simulink model "Model_Platform"  (R2018a)
settings: Solver=ode1  StartTime=0.0  StopTime=inf  FixedStep=0.001  RelTol=1e-3  EnableMultiTasking=on
PreLoadFcn:
  | ;HLABlocksetInit;;HLABlocksetInit;;HLABlocksetInit;
PostLoadFcn:
  | ;set_param(gcs,'PostCodeGenCommand', 'rtw_defines(buildInfo)');;set_param(gcs,'PostCodeGenCommand', 'rtw_defines(buildInfo)');;set_param(gcs,'PostCodeGenCommand', 'rtw_defines(buildInfo)');
undefined symbols (not defined in the file or in its folder): eng_speed, Heading_init, inertiaLateral, Joystick, Newton, omega_engine, omega_max, omega_wheel, Para, radiusWheel, Raphson, Standard_Devices, torque, Torque_lost, Torque_lost_wheel, X_init, Y_init, Z_init
libraries: simulink x26, dspnetwork x4, rtwinlib x2, PC_Simulator_Lib x2, vrlib x1
(part 1 of 4)
settings Model: ExtModeTrigDuration=1000001  Creator=Mohamed  LastModifiedBy=mario.franke
settings DataIOCC: LimitDataPoints=on  SaveFormat=Array  SignalLoggingSaveFormat=ModelDataLogs  ReturnWorkspaceOutputs=on
settings OptimizationCC: ExpressionDepthLimit=2147483647  LifeSpan=inf
settings DebuggingCC: ReadBeforeWriteMsg=DisableAll  WriteAfterWriteMsg=DisableAll  WriteAfterReadMsg=DisableAll  UnderspecifiedInitializationDetection=Classic  MergeDetectMultiDrivingBlocksExec=none  SolverPrmCheckMsg=warning  MultiTaskDSMMsg=none  MultiTaskRateTransMsg=warning  IntegerOverflowMsg=none  StateNameClashWarn=warning  SFUnexpectedBacktrackingDiag=warning  SFNoUnconditionalDefaultTransitionDiag=warning  SFExecutionAtInitializationDiag=none  IntegerSaturationMsg=none
settings HardwareCC: ProdBitPerPointer=32  ProdBitPerSizeT=32  ProdBitPerPtrDiffT=32  ProdLargestAtomicFloat=None  ProdWordSize=32  ProdHWDeviceType=Generic->32-bit x86 compatible
settings ModelReferenceCC: UpdateModelReferenceTargets=IfOutOfDate  PropagateSignalLabelsOutOfModel=off
settings SFSimCC: SFSimEcho=off
settings RTWCC: PostCodeGenCommand=rtw_defines(buildInfo)  Description=Generic Real-Time Target  RTWCompilerOptimization=on
settings CodeAppCC: MaxIdLength=95  StateflowObjectComments=on
settings GRTTargetCC: TargetLangStandard=C89/C90 (ANSI)  GeneratePreprocessorConditionals=Disable all
settings ConfigComp: CovMetricSettings=dw  CovHtmlReporting=on  CovSaveCumulativeToWorkspaceVar=on  CovSaveSingleToWorkspaceVar=on  CovExternalEMLEnable=off
settings SimscapeCC: SimscapeNormalizeSystem=off
settings ConfigurationSet: Description=SimMechanics 2G

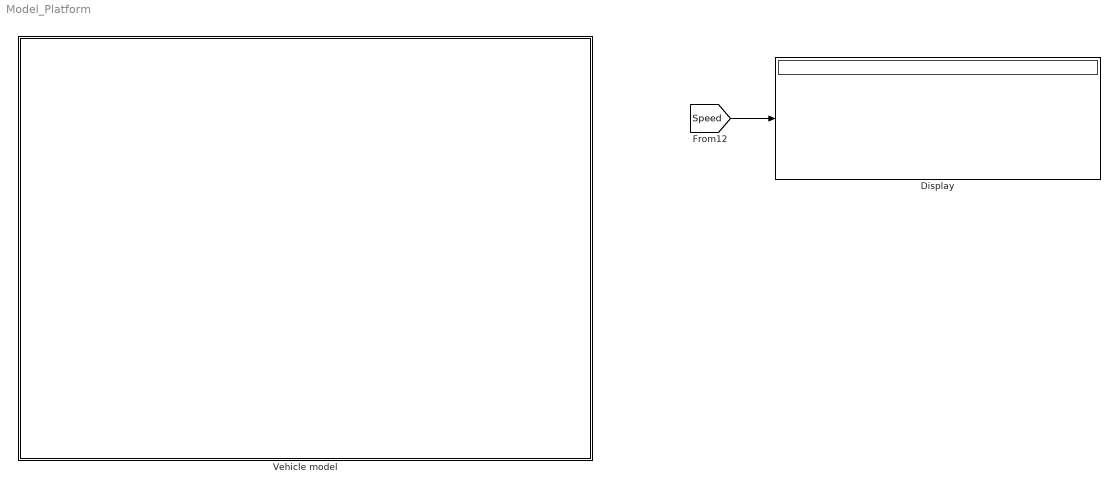
== system Model_Platform ==
  Display : Display
      settings: Format=bank
  Vehicle model : Subsystem
      mask Display: image(imread('Image.jpg'))
  wires:
  [Speed] -> Display/1

== system Model_Platform/Vehicle model ==
  Bus Creator : BusCreator  Inputs=3
  Comunication_with_visualisation_normal_mode1 : Subsystem  AncestorBlock=PC_Simulator_Lib/Comunication_with_visualisation_normal_mode
  Display : Display
      settings: Format=bank
  Drive_Train : Subsystem  AncestorBlock=PC_Simulator_Lib/Drive_Train
  HMI_Realtime_normal_mode : Subsystem  AncestorBlock=PC_Simulator_Lib/HMI_Realtime_normal_mode
  Remaining Computation Time (must be positive) : Scope  Commented=on
  Timer for Real-Time : S-Function  FunctionName=sfun_rttime  Parameters=1  SFunctionDeploymentMode=off  EnableBusSupport=off
  Vehicle dynamics : Subsystem  AncestorBlock=PC_Simulator_Lib/Vehicle dynamics
  wires:
  Drive_Train/1(Drive_Train) -> Bus Creator/2
  Bus Creator/1 -> HMI_Realtime_normal_mode/1(feedback), Drive_Train/1(feedback), Comunication_with_visualisation_normal_mode1/1(FeedBack), Vehicle dynamics/1(Feedback)
  Vehicle dynamics/1(Vehicle_Dynamics) -> Bus Creator/3
  Timer for Real-Time/1 -> Remaining Computation Time (must be positive)/1
  [Speed] -> Display/1
  HMI_Realtime_normal_mode/1(Driver_Interface) -> Bus Creator/1

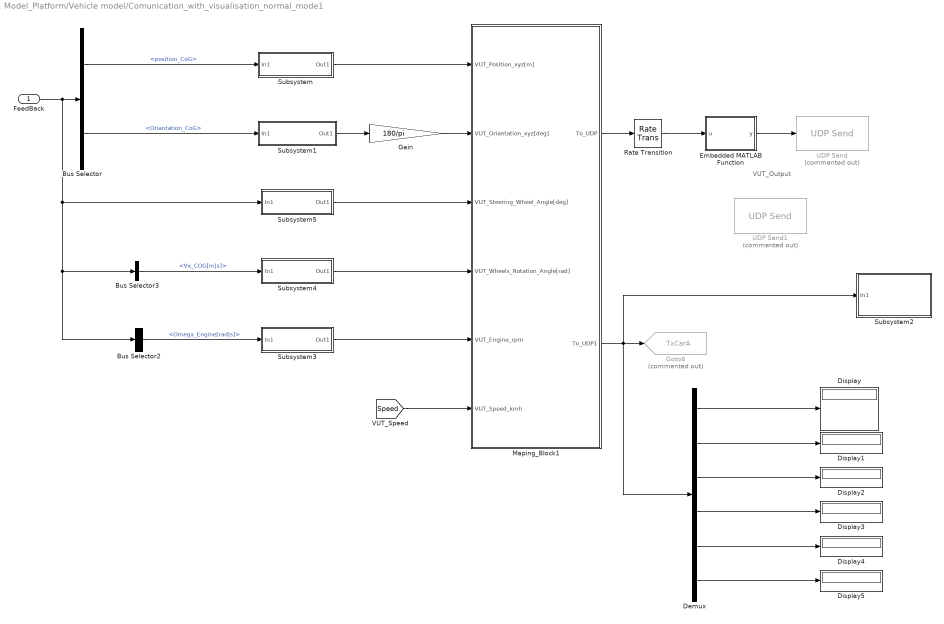
== system Model_Platform/Vehicle model/Comunication_with_visualisation_normal_mode1 ==
  note: VUT_Output
  FeedBack : Inport
  Bus Selector : BusSelector  OutputSignals=Vehicle_Dynamics.position_CoG,Vehicle_Dynamics.Oriantation_CoG
  Bus Selector2 : BusSelector  OutputSignals=Drive_Train.Omega_Engine[rad|s]
  Bus Selector3 : BusSelector  OutputSignals=Vehicle_Dynamics.Vx_COG[m|s]
  Demux : Demux  Outputs=6
  Display{,1..5} (6 alike) : Display
  Embedded MATLAB Function : MATLAB Function  TreatAsAtomicUnit=on
  Gain : Gain  Gain=180/pi
  Goto6 : Goto  Commented=on  GotoTag=TxCarA  TagVisibility=global
  Maping_Block1 : Subsystem
  Rate Transition : RateTransition
  Subsystem : Subsystem
  Subsystem1 : Subsystem
  Subsystem2 : Subsystem  TreatAsAtomicUnit=on  SystemSampleTime=1/20
  Subsystem3 : Subsystem
  Subsystem4 : Subsystem
  Subsystem5 : Subsystem
  UDP Send : dspnetwork/UDP Send  Commented=on  remoteURL='169.254.83.115'  remotePort=15005  localURL='0.0.0.0'  localPortSource=Specify via dialog  localPort=-1  sampletime=-1  blockPlatform=[]  separateLengthPort=0
      settings: SourceProductName=DSP System Toolbox  SourceProductBaseCode=DS
  UDP Send1 : dspnetwork/UDP Send  Commented=on  remoteURL='131.234.86.53'  remotePort=14000  localURL='0.0.0.0'  localPortSource=Specify via dialog  localPort=-1  sampletime=-1  blockPlatform=[]  separateLengthPort=0
      settings: SourceProductName=DSP System Toolbox  SourceProductBaseCode=DS
  wires:
  Embedded MATLAB Function/1(y) -> UDP Send/1
  Bus Selector/2 -> Subsystem1/1(In1)  "<Oriantation_CoG>"
  Bus Selector/1 -> Subsystem/1(In1)  "<position_CoG>"
  Subsystem1/1(Out1) -> Gain/1
  Gain/1 -> Maping_Block1/2(VUT_Oriantation_xyz[deg])
  Maping_Block1/1(To_UDP) -> Rate Transition/1
  Subsystem3/1(Out1) -> Maping_Block1/5(VUT_Engine_rpm)
  Bus Selector3/1 -> Subsystem4/1(In1)  "<Vx_COG[m|s]>"
  Subsystem4/1(Out1) -> Maping_Block1/4(VUT_Wheels_Rotation_Angle[rad])
  FeedBack/1 -> Bus Selector2/1, Bus Selector3/1, Subsystem5/1(In1), Bus Selector/1
  Bus Selector2/1 -> Subsystem3/1(In1)  "<Omega_Engine[rad|s]>"
  Subsystem/1(Out1) -> Maping_Block1/1(VUT_Position_xyz[m])
  Subsystem5/1(Out1) -> Maping_Block1/3(VUT_Steering_Wheel_Angle[deg])
  [Speed] -> Maping_Block1/6(VUT_Speed_kmh)
  Demux/3 -> Display2/1
  Demux/2 -> Display1/1
  Demux/1 -> Display/1
  Demux/6 -> Display5/1
  Demux/5 -> Display4/1
  Demux/4 -> Display3/1
  Rate Transition/1 -> Embedded MATLAB Function/1(u)
  Maping_Block1/2(To_UDP1) -> Subsystem2/1(In1), Demux/1, Goto6/1

== system Model_Platform/Vehicle model/Drive_Train ==
  feedback : Inport
  4_Wheels_drive_train_and_Brake : Subsystem
  Bus Selector : BusSelector  OutputSignals=Vehicle_Dynamics.Vx_COG[m|s],Driver_Interface.DNR
  Bus Selector1 : BusSelector  OutputSignals=Driver_Interface.Acc_Pedal_norm
  Differential : Subsystem
  Engine : Subsystem
  Gain : Gain  Gain=3.6
  Gearbox : Subsystem
  Mux2 : Mux  Inputs=2
  Mux3 : Mux  Inputs=2
  Output_Interface : Subsystem
  Drive_Train : Outport
  wires:
  Bus Selector1/1 -> Engine/1(Throttle)  "<Acc_Pedal_norm>"
  Gearbox/4(Gearbox_Gear_Ratio) -> Output_Interface/14(Gearbox_Gear_Ratio)
  4_Wheels_drive_train_and_Brake/10(Omega_FR[rad|s]) -> Output_Interface/10(Omega_FR[rad|s])
  4_Wheels_drive_train_and_Brake/9(Omega_FL[rad|s]) -> Output_Interface/9(Omega_FL[rad|s])
  4_Wheels_drive_train_and_Brake/8(Fy_RR[N]) -> Output_Interface/8(Force_tire_y_RR[N])  "Force_tire_y_RR_N"
  4_Wheels_drive_train_and_Brake/7(Fy_RL[N]) -> Output_Interface/7(Force_tire_y_RL[N])  "Force_tire_y_RL_N"
  4_Wheels_drive_train_and_Brake/6(Fy_FR[N]) -> Output_Interface/6(Force_tire_y_FR[N])  "Force_tire_y_FR_N"
  4_Wheels_drive_train_and_Brake/5(Fy_FL[N]) -> Output_Interface/5(Force_tire_y_FL[N])  "Force_tire_y_FL_N"
  4_Wheels_drive_train_and_Brake/4(Fx_RR[N]) -> Output_Interface/4(Force_tire_x_RR[N])
  4_Wheels_drive_train_and_Brake/3(Fx_RL[N]) -> Output_Interface/3(Force_tire_x_RL[N])
  4_Wheels_drive_train_and_Brake/2(Fx_FR[N]) -> Output_Interface/2(Force_tire_x_FR[N])
  4_Wheels_drive_train_and_Brake/1(Fx_FL[N]) -> Output_Interface/1(Force_tire_x_FL[N])
  Gearbox/3(omegaDot_engine_radPs2) -> Engine/3(OmegaDot_engine_radPs2)
  Mux3/1 -> Differential/3(rotation_2)
  Mux2/1 -> Differential/2(rotation_1)
  4_Wheels_drive_train_and_Brake/14(OmegaDot_RR[rad|s^2]) -> Mux3/2
  4_Wheels_drive_train_and_Brake/13(Omega_RR[rad|s]) -> Output_Interface/12(Omega_RR[rad|s]), Mux3/1
  4_Wheels_drive_train_and_Brake/12(OmegaDot_RL[rad|s^2]) -> Mux2/2
  4_Wheels_drive_train_and_Brake/11(Omega_RL[rad|s]) -> Output_Interface/11(Omega_RL[rad|s]), Mux2/1
  Differential/2(Torque_out_2) -> 4_Wheels_drive_train_and_Brake/3(Torque_RR[Nm])
  Differential/1(Torque_out_1) -> 4_Wheels_drive_train_and_Brake/2(Torque_RL[Nm])
  Differential/4(omegaDot_out_gearbox_radPs1) -> Gearbox/5(omegaDot_out_gearbox_radPs2)
  Differential/3(omega_out_gearbox_radPs) -> Gearbox/4(omega_out_gearbox_radPs)
  Gearbox/2(Torque_out_gearbox_Nm) -> Differential/1(Torque_in)
  Gearbox/1(omega_engine_radPs) -> Output_Interface/13(Omega_Engine[rad|s]), Engine/2(Omega_engine_radPs)
  Engine/1(Torque) -> Gearbox/3(Torque_Engine)
  Bus Selector/2 -> Gearbox/2(DNR)  "<DNR>"
  Gain/1 -> Gearbox/1(velocity)
  Bus Selector/1 -> Gain/1  "<Vx_COG[m|s]>"
  feedback/1 -> Bus Selector1/1, Bus Selector/1, 4_Wheels_drive_train_and_Brake/1(Feedback)
  Output_Interface/1(Drive_Train) -> Drive_Train/1

== system Model_Platform/Vehicle model/HMI_Realtime_normal_mode ==
  note: D..1
      | N..0
      | R..-1
  feedback : Inport
  Bus Selector : BusSelector  Commented=on  OutputSignals=ADAS.Steering_Wheel_Angle[norm]
  Bus Selector1 : BusSelector  Commented=on  OutputSignals=ADAS.Enable_Lateral_Controller
  Gain3 : Gain  Commented=on  Gain=450
  Gain4 : Gain  Commented=on  Gain=450
  HMI_Logitech1 : Subsystem  AncestorBlock=PC_Simulator_Lib/HMI_Realtime/HMI_Logitech1
  Maping_Output : PC_Simulator_Lib/HMI_Realtime/Maping_Output
  Terminator{3..7} (5 alike) : Terminator
  steering wheel controller : PC_Simulator_Lib/HMI_Realtime/steering wheel controller  Commented=on
  Driver_Interface : Outport
  wires:
  Bus Selector1/1 -> steering wheel controller/3  "<Enable_Lateral_Controller>"
  HMI_Logitech1/11(Button_6) -> Maping_Output/11
  steering wheel controller/1 -> HMI_Logitech1/1(Force_Feedback)
  HMI_Logitech1/16(arrow_deg) -> Terminator7/1
  HMI_Logitech1/15(Button_10) -> Terminator6/1
  HMI_Logitech1/14(Button_9) -> Terminator5/1
  HMI_Logitech1/13(Button_8) -> Terminator4/1
  HMI_Logitech1/12(Button_7) -> Terminator3/1
  HMI_Logitech1/8(Right_Padel) -> Maping_Output/8
  HMI_Logitech1/9(Left_Padel) -> Maping_Output/9
  HMI_Logitech1/10(Button_5) -> Maping_Output/10
  Maping_Output/1 -> Driver_Interface/1
  HMI_Logitech1/17(DNR) -> Maping_Output/12  "DNR"
  HMI_Logitech1/7(Button_4) -> Maping_Output/7
  HMI_Logitech1/6(Button_3) -> Maping_Output/6
  HMI_Logitech1/5(Button_2) -> Maping_Output/5
  HMI_Logitech1/4(Button_1) -> Maping_Output/4
  Bus Selector/1 -> Gain3/1  "<Steering_Wheel_Angle[norm]>"
  feedback/1 -> Bus Selector1/1, Bus Selector/1
  Gain3/1 -> steering wheel controller/2
  Gain4/1 -> steering wheel controller/1
  HMI_Logitech1/1(Steering_Wheel_norm) -> Maping_Output/1, Gain4/1  "Steering_wheel_norm"
  HMI_Logitech1/2(Acceleration_pedal) -> Maping_Output/2  "Acc_Pedal_norm"
  HMI_Logitech1/3(Brack_pedal) -> Maping_Output/3  "Brake_Pedal_norm"

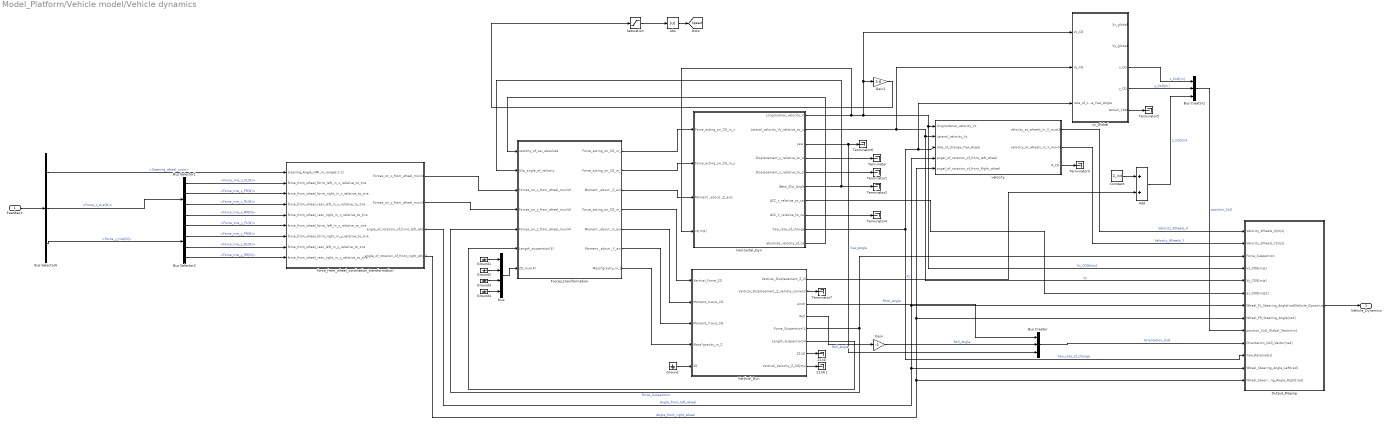
== system Model_Platform/Vehicle model/Vehicle dynamics ==
  Feedback : Inport
  Abs : Abs
  Add : Sum
  Bus Creator : BusCreator  Inputs=3
  Bus Creator1 : BusCreator  Inputs=3
  Bus Selector1 : BusSelector  OutputSignals=Force_tire_x_FL[N],Force_tire_x_FR[N],Force_tire_x_RL[N],Force_tire_x_RR[N]
  Bus Selector2 : BusSelector  OutputSignals=Force_tire_y_FL[N],Force_tire_y_FR[N],Force_tire_y_RL[N],Force_tire_y_RR[N]
  Bus Selector6 : BusSelector  OutputSignals=Driver_Interface.Steering_wheel_norm,Drive_Train.Force_x_tire[N],Drive_Train.Force_y_tire[N]
  Constant : Constant  Value=Z_init
  Forces_transformation : Subsystem
  Gain : Gain  Gain=-1
  Gain1 : Gain  Gain=3.6
  Ground{,1..4} (5 alike) : Ground
  Horizontal_Dyn : Subsystem
  Mux : Mux
  Output_Maping : Subsystem
  Saturation : Saturate  UpperLimit=180  LowerLimit=-180
  Terminator{,1..7} (8 alike) : Terminator
  Vertical_Dyn. : Subsystem
  Z1(4) : Terminator
  Z1(4)1 : Terminator
  force_from_wheel_cordination_transformation : Subsystem
  velocity : Subsystem
  xy_Global : Subsystem
  Vehicle_Dynamics : Outport
  tag scope: Speed=global
  wires:
  xy_Global/5(Actual_YAW) -> Terminator5/1
  Ground4/1 -> Mux/4
  Ground3/1 -> Mux/3
  Ground2/1 -> Mux/2
  Ground1/1 -> Mux/1
  Mux/1 -> Forces_transformation/7(Z0_mux(4))
  Ground/1 -> Vertical_Dyn./5(Z0)
  Vertical_Dyn./8(Vertical_Velocity_Z_CG[m|s]) -> Z1(4)1/1
  velocity/3(R_CG) -> Terminator3/1
  Bus Selector2/4 -> force_from_wheel_cordination_transformation/9(force_from_wheel_rear_right_in_y_relative_to_tire)  "<Force_tire_y_RR[N]>"
  Bus Selector2/3 -> force_from_wheel_cordination_transformation/8(force_from_wheel_rear_left_in_y_relative_to_tire)  "<Force_tire_y_RL[N]>"
  Bus Selector2/2 -> force_from_wheel_cordination_transformation/7(force_from_wheel_fornt_right_in_y_relative_to_tire)  "<Force_tire_y_FR[N]>"
  Bus Selector2/1 -> force_from_wheel_cordination_transformation/6(force_from_wheel_fornt_left_in_y_relative_to_tire)  "<Force_tire_y_FL[N]>"
  Bus Selector6/3 -> Bus Selector2/1  "<Force_y_tire[N]>"
  Bus Creator/1 -> Output_Maping/10(Oriantation_CoG_Vector[rad])  "Oriantation_CoG"
  Bus Creator1/1 -> Output_Maping/9(position_CoG_Global_Vector[m])  "position_CoG"
  Constant/1 -> Add/1
  Add/1 -> Bus Creator1/3  "z_CoG[m]"
  Vertical_Dyn./1(Vertical_Displacement_Z_CG) -> Add/2  "Vz"
  Output_Maping/1(Vehicle_Dynamics) -> Vehicle_Dynamics/1
  xy_Global/4(y_CG) -> Bus Creator1/2  "y_CoG[m]"
  xy_Global/3(x_CG) -> Bus Creator1/1  "x_CoG[m]"
  Bus Selector6/1 -> force_from_wheel_cordination_transformation/1(steering_Angle_HMI_in_range[-1 1])  "<Steering_wheel_norm>"
  Gain1/1 -> Saturation/1
  Bus Selector6/2 -> Bus Selector1/1  "<Force_x_tire[N]>"
  Feedback/1 -> Bus Selector6/1
  Horizontal_Dyn/3("yaw ") -> Terminator6/1, Bus Creator/3  "Yaw_Angle"
  Forces_transformation/7(Mass*gravity_in_Z) -> Vertical_Dyn./4(Mass*gravity_in_Z)
  velocity/2(velocity_at_wheels_in_Y_mux(4)) -> Output_Maping/2(Velocity_Wheels_Y[m|s])  "Velocity_Wheels_Y"
  velocity/1(velocity_at_wheels_in_X_mux(4)) -> Output_Maping/1(Velocity_Wheels_X[m|s])  "Velocity_Wheels_X"
  Vertical_Dyn./7(Z1(4)) -> Z1(4)/1
  Vertical_Dyn./2(Vertical_Displacement_Z_vehicle_corners(4)) -> Terminator7/1
  Vertical_Dyn./4(Roll) -> Gain/1  "Roll_Angle"
  Vertical_Dyn./3(pitch) -> Bus Creator/1  "Pitch_Angle"
  Bus Selector1/4 -> force_from_wheel_cordination_transformation/5(force_from_wheel_rear_right_in_x_relative_to_tire)  "<Force_tire_x_RR[N]>"
  Bus Selector1/3 -> force_from_wheel_cordination_transformation/4(force_from_wheel_rear_left_in_x_relative_to_tire)  "<Force_tire_x_RL[N]>"
  Bus Selector1/2 -> force_from_wheel_cordination_transformation/3(force_from_wheel_fornt_right_in_x_relative_to_tire)  "<Force_tire_x_FR[N]>"
  Bus Selector1/1 -> force_from_wheel_cordination_transformation/2(force_from_wheel_fornt_left_in_x_relative_to_tire)  "<Force_tire_x_FL[N]>"
  Vertical_Dyn./6(Length_Suspention(4)) -> Forces_transformation/6(Length_suspention(4))
  Forces_transformation/6(Moment _about _Y_axis) -> Vertical_Dyn./3(Moment_Y-axis_CG)
  Forces_transformation/5(Moment _about _X_axis) -> Vertical_Dyn./2(Moment_X-axis_CG)
  Forces_transformation/4(Force_acting_on_CG_in_z) -> Vertical_Dyn./1(Vertical_Force_CG)
  Forces_transformation/3(Moment _about _Z_axis) -> Horizontal_Dyn/3(Moment _about _Z_axis)
  Forces_transformation/2(Force_acting_on_CG_in_Y) -> Horizontal_Dyn/2(Force_acting_on_CG_in_y)
  Forces_transformation/1(Force_acting_on_CG_in_x) -> Horizontal_Dyn/1(Force_acting_on_CG_in_x)
  Vertical_Dyn./5(Force_Suspention(4)) -> Output_Maping/3(Force_Suspention), Forces_transformation/5(Forces_on_z_from_wheel_mux(4))  "Force_Suspention"
  force_from_wheel_cordination_transformation/2(Forces_on_y_from_wheel_mux(4)) -> Forces_transformation/4(Forces_on_y_from_wheel_mux(4))
  force_from_wheel_cordination_transformation/1(Forces_on_x_from_wheel_mux(4)) -> Forces_transformation/3(Forces_on_x_from_wheel_mux(4))
  Horizontal_Dyn/10(absolute_velocity_of_car) -> Forces_transformation/1(velocity_of_car_absolute)
  force_from_wheel_cordination_transformation/4(angle_of_rotation_of_front_right_wheel) -> Output_Maping/8(Wheel_FR_Steering_Angle[rad]), velocity/5(angel_of_rotation_of_front_Right_wheel), Output_Maping/13(Wheel_Steering_Angle_Right[rad])  "Angle_front_right_wheel"
  force_from_wheel_cordination_transformation/3(angle_of_rotation_of_front_left_wheel) -> Output_Maping/7(Wheel_FL_Steering_Angle[rad]), velocity/4(angel_of_rotation_of_front_left_wheel), Output_Maping/12(Wheel_Steering_Angle_Left[rad])  "Angle_front_left_wheel"
  Horizontal_Dyn/9(Yaw_rate_of_change) -> xy_Global/3(rate_of_change_Yaw_Angle), velocity/3(rate_of_change_Yaw_Angle), Output_Maping/11(Yaw_Rate[rad|s])  "Yaw_rate_of_change"
  Horizontal_Dyn/8(ACC_Y_relative_to_car) -> Terminator4/1
  Horizontal_Dyn/7(ACC_x_relative_to_car) -> Output_Maping/6(ax_COG[m|s2])
  Horizontal_Dyn/4(Displacement_y_relative_to_car) -> Terminator/1
  Horizontal_Dyn/5(Displacement_x_relative_to_car) -> Terminator1/1
  Horizontal_Dyn/6(Beta_Slip_Angle) -> Forces_transformation/2(Slip_angle_of_velocity), Terminator2/1
  Horizontal_Dyn/2(Lateral_velocity_Vy_relative_to_car) -> velocity/2(Lateral_velocity_Vy), Output_Maping/5(Vy_COG[m|s]), xy_Global/2(Vy_CG)  "Vy"
  Horizontal_Dyn/1(Longitudinal_velocity_Vx) -> xy_Global/1(Vx_CG), Gain1/1, Output_Maping/4(Vx_COG[m|s]), velocity/1(longitudenal_velocity_Vx), Horizontal_Dyn/4(vx[m|s])  "Vx_COG[m|s]"
  Saturation/1 -> Abs/1
  Abs/1 -> [Speed]
  Gain/1 -> Bus Creator/2  "Roll_Angle"

== system Model_Platform/Vehicle model/Comunication_with_visualisation_normal_mode1/Maping_Block1 ==
  note: Gamma_2nd_Car
  note: z_2nd_Car
  note: y_2nd_Car
  note: x_2nd_Car
  VUT_Position_xyz[m] : Inport
  VUT_Oriantation_xyz[deg] : Inport  Port=2
  VUT_Steering_Wheel_Angle[deg] : Inport  Port=3
  VUT_Wheels_Rotation_Angle[rad] : Inport  Port=4
  VUT_Engine_rpm : Inport  Port=5
  VUT_Speed_kmh : Inport  Port=6
  Add : Sum
  Demux : Demux  Outputs=6
  Display : Display
  Dummy_value : Constant  Value=0
  Dummy_value1 : Constant  Value=.01
  Gain1 : Gain  Gain=2.5
  Mux : Mux  Inputs=12
  Mux1 : Mux
  Terminator : Terminator
  Terminator1 : Terminator
  UDP Receive : dspnetwork/UDP Receive  Commented=on  localURL='0.0.0.0'  localPort=15006  remoteURL='192.168.2.103'  remotePort=-1  recvBufferSize=24  dims=6  signalDatatype=double  isVarSize=off  showBlockingTime=off  blockingTime=0  sampletime=0.05  blockPlatform=[]
      settings: SourceProductName=DSP System Toolbox  SourceProductBaseCode=DS
  WheelRot_second_car : Constant  Value=2
  To_UDP : Outport
  To_UDP1 : Outport  Port=2
  wires:
  VUT_Position_xyz[m]/1 -> Mux/1, Mux1/1
  VUT_Oriantation_xyz[deg]/1 -> Mux1/2, Mux/2
  Mux1/1 -> To_UDP1/1
  VUT_Steering_Wheel_Angle[deg]/1 -> Gain1/1
  Gain1/1 -> Mux1/3, Display/1, Mux/3
  Mux/1 -> To_UDP/1
  Demux/6 -> Mux/9
  WheelRot_second_car/1 -> Mux/10
  VUT_Engine_rpm/1 -> Mux/11
  VUT_Speed_kmh/1 -> Mux1/4, Mux/12
  Demux/5 -> Terminator/1
  Demux/4 -> Terminator1/1
  UDP Receive/1 -> Demux/1
  VUT_Wheels_Rotation_Angle[rad]/1 -> Mux/5
  Dummy_value/1 -> Mux/4
  Demux/2 -> Mux/7
  Demux/3 -> Add/1
  Add/1 -> Mux/8
  Dummy_value1/1 -> Add/2
  Demux/1 -> Mux/6

== system Model_Platform/Vehicle model/Comunication_with_visualisation_normal_mode1/Subsystem ==
  In1 : Inport
  Bus Selector : BusSelector  OutputSignals=x_CoG[m],y_CoG[m],z_CoG[m]
  Mux : Mux  Inputs=3
  Out1 : Outport
  wires:
  In1/1 -> Bus Selector/1
  Mux/1 -> Out1/1
  Bus Selector/3 -> Mux/3  "<z_CoG[m]>"
  Bus Selector/2 -> Mux/2  "<y_CoG[m]>"
  Bus Selector/1 -> Mux/1  "<x_CoG[m]>"

== system Model_Platform/Vehicle model/Comunication_with_visualisation_normal_mode1/Subsystem1 ==
  In1 : Inport
  Bus Selector : BusSelector  OutputSignals=Pitch_Angle,Roll_Angle,Yaw_Angle
  Mux : Mux  Inputs=3
  Saturation : Saturate  UpperLimit=0.15  LowerLimit=-0.14
  Out1 : Outport
  wires:
  Bus Selector/1 -> Saturation/1  "<Pitch_Angle>"
  Bus Selector/2 -> Mux/2  "<Roll_Angle>"
  Bus Selector/3 -> Mux/3  "<Yaw_Angle>"
  Mux/1 -> Out1/1
  In1/1 -> Bus Selector/1
  Saturation/1 -> Mux/1

== system Model_Platform/Vehicle model/Comunication_with_visualisation_normal_mode1/Subsystem2 ==
  In1 : Inport
  UDP Send : dspnetwork/UDP Send  remoteURL='192.168.1.118'  remotePort=15006  localURL='0.0.0.0'  localPortSource=Automatically determine  localPort=-1  sampletime=-1  blockPlatform=[]  separateLengthPort=0
      settings: SourceProductName=DSP System Toolbox  SourceProductBaseCode=DS
  wires:
  In1/1 -> UDP Send/1

== system Model_Platform/Vehicle model/Comunication_with_visualisation_normal_mode1/Subsystem3 ==
  In1 : Inport
  Add : Sum
  Constant : Constant  Value=1000
  Gain1 : Gain  Gain=60/(2*pi)
  Out1 : Outport
  wires:
  In1/1 -> Gain1/1
  Add/1 -> Out1/1
  Gain1/1 -> Add/1
  Constant/1 -> Add/2

== system Model_Platform/Vehicle model/Comunication_with_visualisation_normal_mode1/Subsystem4 ==
  In1 : Inport
  Gain : Gain  Gain=1/radiusWheel
  Integrator : Integrator
  Out1 : Outport
  wires:
  Integrator/1 -> Out1/1
  In1/1 -> Gain/1
  Gain/1 -> Integrator/1

== system Model_Platform/Vehicle model/Comunication_with_visualisation_normal_mode1/Subsystem5 ==
  In1 : Inport
  Add : Sum
  Bus Selector3 : BusSelector  OutputSignals=Vehicle_Dynamics.Wheel_Steering_Angle_Left[rad],Vehicle_Dynamics.Wheel_Steering_Angle_Right[rad]
  Gain : Gain  Gain=-0.5
  Gain1 : Gain  Gain=180/pi
  Out1 : Outport
  wires:
  In1/1 -> Bus Selector3/1
  Bus Selector3/1 -> Add/1  "<Wheel_Steering_Angle_Left[rad]>"
  Bus Selector3/2 -> Add/2  "<Wheel_Steering_Angle_Right[rad]>"
  Add/1 -> Gain/1
  Gain/1 -> Gain1/1
  Gain1/1 -> Out1/1

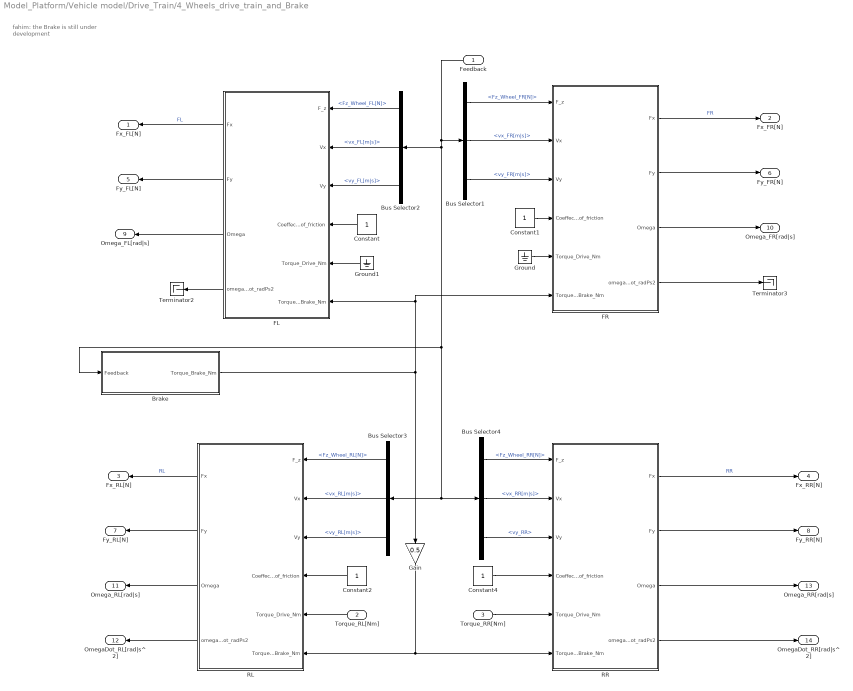
== system Model_Platform/Vehicle model/Drive_Train/4_Wheels_drive_train_and_Brake ==
  note: fahim:
      | the Brake is still under development
  Feedback : Inport
  Torque_RL[Nm] : Inport  Port=2
  Torque_RR[Nm] : Inport  Port=3
  Brake : Subsystem
  Bus Selector1 : BusSelector  OutputSignals=Vehicle_Dynamics.Fz_Wheel.Fz_Wheel_FR[N],Vehicle_Dynamics.Velocity_Wheels[m|s].v_FR[m|s].vx_FR[m|s],Vehicle_Dynamics.Velocity_Wheels[m|s].v_FR[m|s].vy_FR[m|s]
  Bus Selector2 : BusSelector  OutputSignals=Vehicle_Dynamics.Fz_Wheel.Fz_Wheel_FL[N],Vehicle_Dynamics.Velocity_Wheels[m|s].v_FL[m|s].vx_FL[m|s],Vehicle_Dynamics.Velocity_Wheels[m|s].v_FL[m|s].vy_FL[m|s]
  Bus Selector3 : BusSelector  OutputSignals=Vehicle_Dynamics.Fz_Wheel.Fz_Wheel_RL[N],Vehicle_Dynamics.Velocity_Wheels[m|s].v_RL[m|s].vx_RL[m|s],Vehicle_Dynamics.Velocity_Wheels[m|s].v_RL[m|s].vy_RL[m|s]
  Bus Selector4 : BusSelector  OutputSignals=Vehicle_Dynamics.Fz_Wheel.Fz_Wheel_RR[N],Vehicle_Dynamics.Velocity_Wheels[m|s].v_RR[m|s].vx_RR[m|s],Vehicle_Dynamics.Velocity_Wheels[m|s].v_RR[m|s].vy_RR
  Constant{,1..2,4} (4 alike) : Constant
  FL : Subsystem
  FR : Subsystem
  Gain : Gain  Gain=0.5
  Ground : Ground
  Ground1 : Ground
  RL : Subsystem
  RR : Subsystem
  Terminator2 : Terminator
  Terminator3 : Terminator
  Fx_FL[N] : Outport
  Fx_FR[N] : Outport  Port=2
  Fx_RL[N] : Outport  Port=3
  Fx_RR[N] : Outport  Port=4
  Fy_FL[N] : Outport  Port=5
  Fy_FR[N] : Outport  Port=6
  Fy_RL[N] : Outport  Port=7
  Fy_RR[N] : Outport  Port=8
  Omega_FL[rad|s] : Outport  Port=9
  Omega_FR[rad|s] : Outport  Port=10
  Omega_RL[rad|s] : Outport  Port=11
  OmegaDot_RL[rad|s^2] : Outport  Port=12
  Omega_RR[rad|s] : Outport  Port=13
  OmegaDot_RR[rad|s^2] : Outport  Port=14
  wires:
  FR/4(omegaDot_radPs2) -> Terminator3/1
  FL/4(omegaDot_radPs2) -> Terminator2/1
  Ground1/1 -> FL/5(Torque_Drive_Nm)
  Ground/1 -> FR/5(Torque_Drive_Nm)
  Gain/1 -> RR/6(Torque_Brake_Nm), RL/6(Torque_Brake_Nm)
  Torque_RR[Nm]/1 -> RR/5(Torque_Drive_Nm)
  Brake/1(Torque_Brake_Nm) -> FR/6(Torque_Brake_Nm), FL/6(Torque_Brake_Nm), Gain/1
  Torque_RL[Nm]/1 -> RL/5(Torque_Drive_Nm)
  FL/3(Omega) -> Omega_FL[rad|s]/1
  FR/3(Omega) -> Omega_FR[rad|s]/1
  RL/4(omegaDot_radPs2) -> OmegaDot_RL[rad|s^2]/1
  RR/4(omegaDot_radPs2) -> OmegaDot_RR[rad|s^2]/1
  RR/2(Fy) -> Fy_RR[N]/1
  Constant4/1 -> RR/4(Coeffecient_of_friction)
  Bus Selector4/3 -> RR/3(Vy)  "<vy_RR>"
  Bus Selector4/2 -> RR/2(Vx)  "<vx_RR[m|s]>"
  Bus Selector4/1 -> RR/1(F_z)  "<Fz_Wheel_RR[N]>"
  Bus Selector3/3 -> RL/3(Vy)  "<vy_RL[m|s]>"
  Bus Selector3/2 -> RL/2(Vx)  "<vx_RL[m|s]>"
  Bus Selector3/1 -> RL/1(F_z)  "<Fz_Wheel_RL[N]>"
  Constant2/1 -> RL/4(Coeffecient_of_friction)
  Bus Selector1/3 -> FR/3(Vy)  "<vy_FR[m|s]>"
  Bus Selector1/2 -> FR/2(Vx)  "<vx_FR[m|s]>"
  Bus Selector1/1 -> FR/1(F_z)  "<Fz_Wheel_FR[N]>"
  Constant1/1 -> FR/4(Coeffecient_of_friction)
  Constant/1 -> FL/4(Coeffecient_of_friction)
  Bus Selector2/3 -> FL/3(Vy)  "<vy_FL[m|s]>"
  Bus Selector2/2 -> FL/2(Vx)  "<vx_FL[m|s]>"
  Bus Selector2/1 -> FL/1(F_z)  "<Fz_Wheel_FL[N]>"
  Feedback/1 -> Bus Selector1/1, Bus Selector2/1, Brake/1(Feedback), Bus Selector4/1, Bus Selector3/1
  FL/1(Fx) -> Fx_FL[N]/1  "FL"
  FR/1(Fx) -> Fx_FR[N]/1  "FR"
  RL/3(Omega) -> Omega_RL[rad|s]/1
  RR/3(Omega) -> Omega_RR[rad|s]/1
  RL/1(Fx) -> Fx_RL[N]/1  "RL"
  RR/1(Fx) -> Fx_RR[N]/1  "RR"
  FR/2(Fy) -> Fy_FR[N]/1
  FL/2(Fy) -> Fy_FL[N]/1
  RL/2(Fy) -> Fy_RL[N]/1

== system Model_Platform/Vehicle model/Drive_Train/Differential ==
  Torque_in : Inport
  rotation_1 : Inport  Port=2
  rotation_2 : Inport  Port=3
  Add : Sum
  Add1 : Sum
  Demux : Demux  Outputs=2
  Demux1 : Demux  Outputs=2
  Gain : Gain  Gain=0.5
  Gain1 : Gain  Gain=0.5
  Gain2 : Gain  Gain=0.5
  Ground : Ground
  Memory : Memory
  Subtract1 : Sum  Inputs=+-
  Terminator : Terminator
  moment_of_inertia1 : Gain  Gain=inertiaLateral
  uebersetzung : Gain  Gain=Para.DT.Differential_Gear_ratio.v
  uebersetzung1 : Gain  Gain=Para.DT.Differential_Gear_ratio.v
  uebersetzung2 : Gain  Gain=Para.DT.Differential_Gear_ratio.v
  Torque_out_1 : Outport
  Torque_out_2 : Outport  Port=2
  omega_out_gearbox_radPs : Outport  Port=3
  omegaDot_out_gearbox_radPs1 : Outport  Port=4
  wires:
  Ground/1 -> Subtract1/2
  moment_of_inertia1/1 -> Terminator/1
  Memory/1 -> moment_of_inertia1/1
  Subtract1/1 -> Gain1/1
  uebersetzung2/1 -> omegaDot_out_gearbox_radPs1/1
  uebersetzung1/1 -> Subtract1/1
  Demux1/2 -> Add1/2
  Demux/2 -> Add1/1
  Gain2/1 -> Memory/1, uebersetzung2/1
  Add1/1 -> Gain2/1
  Demux1/1 -> Add/2
  Demux/1 -> Add/1
  rotation_2/1 -> Demux1/1
  rotation_1/1 -> Demux/1
  Gain1/1 -> Torque_out_2/1, Torque_out_1/1
  uebersetzung/1 -> omega_out_gearbox_radPs/1
  Gain/1 -> uebersetzung/1
  Add/1 -> Gain/1
  Torque_in/1 -> uebersetzung1/1

== system Model_Platform/Vehicle model/Drive_Train/Engine ==
  Throttle : Inport
  Omega_engine_radPs : Inport  Port=2
  OmegaDot_engine_radPs2 : Inport  Port=3
  Compare To Constant : simulink/Logic and Bit Operations/Compare To Constant  relop=<=  const=omega_max  OutDataTypeStr=uint8
  Engine_Map : Lookup_n-D  NumberOfTableDimensions=1  BreakpointsForDimension1=eng_speed  BeginIndexSearchUsingPreviousIndexResult=on  Table=torque  InputSameDT=on
  Gain1 : Gain  Gain=60/(2*pi)
  Ground : Ground
  Memory : Memory
  Product : Product  Inputs=3  RndMeth=Zero
  Saturation : Saturate  UpperLimit=1  LowerLimit=0
  Subtract : Sum  Inputs=+-+
  Terminator : Terminator
  friction : Lookup_n-D  NumberOfTableDimensions=1  BreakpointsForDimension1=omega_engine  BeginIndexSearchUsingPreviousIndexResult=on  Table=Torque_lost  InputSameDT=on
  moment_of_inertia : Gain  Gain=Para.DT.Flywheel_Inertia.v*10
  Torque : Outport
  wires:
  Ground/1 -> Subtract/2
  friction/1 -> Subtract/3
  Memory/1 -> moment_of_inertia/1
  OmegaDot_engine_radPs2/1 -> Memory/1
  Subtract/1 -> Torque/1
  moment_of_inertia/1 -> Terminator/1
  Gain1/1 -> friction/1, Compare To Constant/1, Engine_Map/1
  Compare To Constant/1 -> Product/3
  Product/1 -> Subtract/1
  Omega_engine_radPs/1 -> Gain1/1
  Engine_Map/1 -> Product/2
  Saturation/1 -> Product/1
  Throttle/1 -> Saturation/1

== system Model_Platform/Vehicle model/Drive_Train/Gearbox ==
  velocity : Inport
  DNR : Inport  Port=2
  Torque_Engine : Inport  Port=3
  omega_out_gearbox_radPs : Inport  Port=4
  omegaDot_out_gearbox_radPs2 : Inport  Port=5
  Automatic_Gear_box_Controller : Stateflow chart  TreatAsAtomicUnit=on
  Display : Display
  Multiport Switch : MultiPortSwitch  DataPortOrder=Zero-based contiguous  Inputs=7  zeroidx=on
  Product : Product  RndMeth=Zero
  Product1 : Product  RndMeth=Zero
  Product2 : Product  RndMeth=Zero
  Saturation : Saturate  UpperLimit=6  LowerLimit=0
  fifth_gear : Constant  Value=Para.DT.Fifth_Gear_reduction_Ratio.v
  first_gear : Constant  Value=Para.DT.First_Gear_reduction_Ratio.v
  fouth_gear : Constant  Value=Para.DT.Forth_Gear_reduction_Ratio.v
  neutral : Constant  Value=0
  neutral1 : Constant  Value=5000
  reverse : Constant  Value=Para.DT.Reverse_Gear_reduction_Ratio.v
  second_gear : Constant  Value=Para.DT.Second_Gear_reduction_Ratio.v
  third_gear : Constant  Value=Para.DT.Third_Gear_reduction_Ratio.v
  omega_engine_radPs : Outport
  Torque_out_gearbox_Nm : Outport  Port=2
  omegaDot_engine_radPs2 : Outport  Port=3
  Gearbox_Gear_Ratio : Outport  Port=4
  wires:
  reverse/1 -> Multiport Switch/8
  fifth_gear/1 -> Multiport Switch/7
  fouth_gear/1 -> Multiport Switch/6
  third_gear/1 -> Multiport Switch/5
  second_gear/1 -> Multiport Switch/4
  first_gear/1 -> Multiport Switch/3
  Product2/1 -> omegaDot_engine_radPs2/1
  omegaDot_out_gearbox_radPs2/1 -> Product2/2
  omega_out_gearbox_radPs/1 -> Product1/2
  neutral1/1 -> Automatic_Gear_box_Controller/3(omega)
  velocity/1 -> Automatic_Gear_box_Controller/1(velocity)
  neutral/1 -> Multiport Switch/2
  Automatic_Gear_box_Controller/1(gear) -> Display/1, Saturation/1
  Product1/1 -> omega_engine_radPs/1
  Product/1 -> Torque_out_gearbox_Nm/1
  Torque_Engine/1 -> Product/2
  Multiport Switch/1 -> Gearbox_Gear_Ratio/1, Product/1, Product2/1, Product1/1
  Saturation/1 -> Multiport Switch/1
  DNR/1 -> Automatic_Gear_box_Controller/2(DNR)

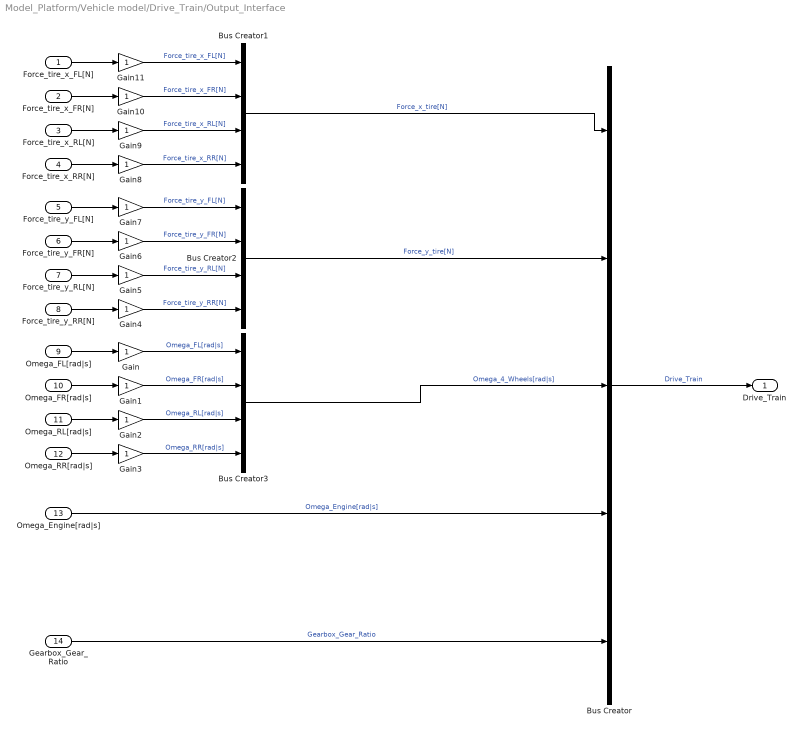
== system Model_Platform/Vehicle model/Drive_Train/Output_Interface ==
  Force_tire_x_FL[N] : Inport
  Force_tire_x_FR[N] : Inport  Port=2
  Force_tire_x_RL[N] : Inport  Port=3
  Force_tire_x_RR[N] : Inport  Port=4
  Force_tire_y_FL[N] : Inport  Port=5
  Force_tire_y_FR[N] : Inport  Port=6
  Force_tire_y_RL[N] : Inport  Port=7
  Force_tire_y_RR[N] : Inport  Port=8
  Omega_FL[rad|s] : Inport  Port=9
  Omega_FR[rad|s] : Inport  Port=10
  Omega_RL[rad|s] : Inport  Port=11
  Omega_RR[rad|s] : Inport  Port=12
  Omega_Engine[rad|s] : Inport  Port=13
  Gearbox_Gear_Ratio : Inport  Port=14
  Bus Creator : BusCreator  Inputs=5
  Bus Creator1 : BusCreator  Inputs=4
  Bus Creator2 : BusCreator  Inputs=4
  Bus Creator3 : BusCreator  Inputs=4
  Gain{,1..11} (12 alike) : Gain
  Drive_Train : Outport
  wires:
  Gearbox_Gear_Ratio/1 -> Bus Creator/5  "Gearbox_Gear_Ratio"
  Omega_Engine[rad|s]/1 -> Bus Creator/4  "Omega_Engine[rad|s]"
  Gain11/1 -> Bus Creator1/1  "Force_tire_x_FL[N]"
  Gain10/1 -> Bus Creator1/2  "Force_tire_x_FR[N]"
  Gain9/1 -> Bus Creator1/3  "Force_tire_x_RL[N]"
  Gain8/1 -> Bus Creator1/4  "Force_tire_x_RR[N]"
  Gain7/1 -> Bus Creator2/1  "Force_tire_y_FL[N]"
  Gain6/1 -> Bus Creator2/2  "Force_tire_y_FR[N]"
  Gain5/1 -> Bus Creator2/3  "Force_tire_y_RL[N]"
  Gain4/1 -> Bus Creator2/4  "Force_tire_y_RR[N]"
  Gain3/1 -> Bus Creator3/4  "Omega_RR[rad|s]"
  Gain2/1 -> Bus Creator3/3  "Omega_RL[rad|s]"
  Gain1/1 -> Bus Creator3/2  "Omega_FR[rad|s]"
  Gain/1 -> Bus Creator3/1  "Omega_FL[rad|s]"
  Bus Creator3/1 -> Bus Creator/3  "Omega_4_Wheels[rad|s]"
  Omega_RR[rad|s]/1 -> Gain3/1
  Omega_RL[rad|s]/1 -> Gain2/1
  Omega_FR[rad|s]/1 -> Gain1/1
  Omega_FL[rad|s]/1 -> Gain/1
  Force_tire_y_RR[N]/1 -> Gain4/1
  Force_tire_y_RL[N]/1 -> Gain5/1
  Force_tire_y_FR[N]/1 -> Gain6/1
  Force_tire_y_FL[N]/1 -> Gain7/1
  Force_tire_x_RR[N]/1 -> Gain8/1
  Bus Creator/1 -> Drive_Train/1  "Drive_Train"
  Force_tire_x_RL[N]/1 -> Gain9/1
  Force_tire_x_FR[N]/1 -> Gain10/1
  Force_tire_x_FL[N]/1 -> Gain11/1
  Bus Creator2/1 -> Bus Creator/2  "Force_y_tire[N]"
  Bus Creator1/1 -> Bus Creator/1  "Force_x_tire[N]"

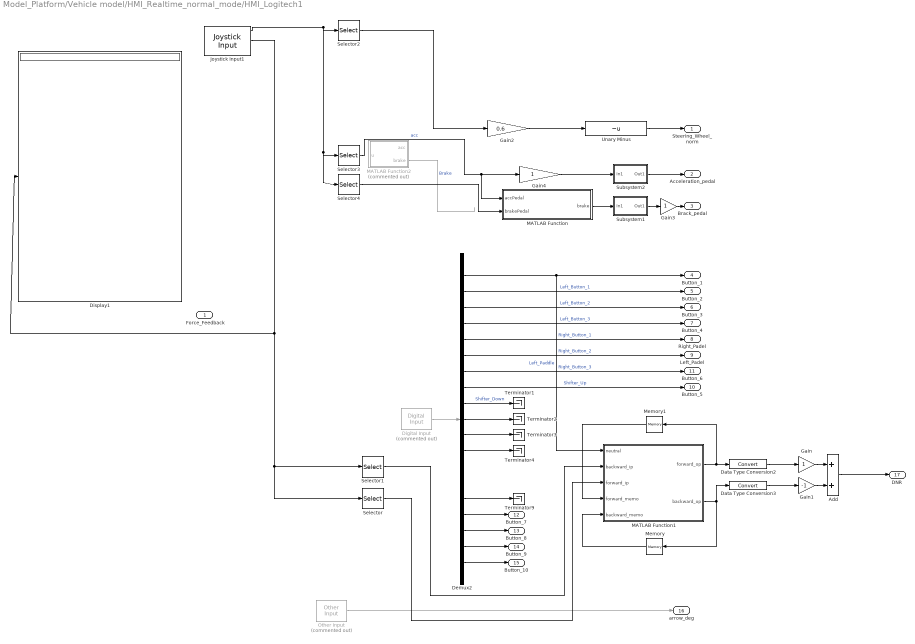
== system Model_Platform/Vehicle model/HMI_Realtime_normal_mode/HMI_Logitech1 ==
  Force_Feedback : Inport
  Add : Sum
  Data Type Conversion2 : DataTypeConversion
  Data Type Conversion3 : DataTypeConversion
  Demux2 : Demux  Outputs=19
  Digital Input : rtwinlib/Digital Input  Commented=on  SampleTime=-1  MaxMissedTicks=inf  ShowMissedTicks=off  YieldWhenWaiting=off  DrvName=Standard_Devices/Joystick  DrvAddress=1  DrvOptions=zeros(1,0)  Channels=1:19  BitMode=2  DataType=1
      settings: AttributesFormatString=Standard Devices\nJoystick [1h]  SourceProductName=Simulink Desktop Real-Time  SourceProductBaseCode=WT
  Display1 : Display
  Gain : Gain
  Gain1 : Gain  Gain=-1
  Gain2 : Gain  Gain=0.6
  Gain3 : Gain
  Gain4 : Gain
  Joystick Input1 : vrlib/Joystick Input  joyid=1  adjustports=on  forcefeed=off
      settings: SourceProductBaseCode=VR
  MATLAB Function : MATLAB Function  TreatAsAtomicUnit=on
  MATLAB Function1 : MATLAB Function  TreatAsAtomicUnit=on
  MATLAB Function2 : MATLAB Function  Commented=on  TreatAsAtomicUnit=on
  Memory : Memory
  Memory1 : Memory
  Other Input : rtwinlib/Other Input  Commented=on  SampleTime=-1  MaxMissedTicks=[]  ShowMissedTicks=off  YieldWhenWaiting=off  DrvName=Standard_Devices/Joystick  DrvAddress=1  DrvOptions=zeros(1,0)  Channels=1  OptParam=0  DataType=1
      settings: AttributesFormatString=Standard Devices\nJoystick [1h]  SourceProductName=Simulink Desktop Real-Time  SourceProductBaseCode=WT
  Selector : Selector  InputPortWidth=21  IndexOptions=Index vector (dialog)  Indices=13  OutputSizes=1
  Selector1 : Selector  InputPortWidth=21  IndexOptions=Index vector (dialog)  Indices=14  OutputSizes=1
  Selector2 : Selector  InputPortWidth=4  IndexOptions=Index vector (dialog)  Indices=1  OutputSizes=1
  Selector3 : Selector  InputPortWidth=4  IndexOptions=Index vector (dialog)  Indices=2  OutputSizes=1
  Selector4 : Selector  InputPortWidth=4  IndexOptions=Index vector (dialog)  Indices=3  OutputSizes=1
  Subsystem1 : Subsystem
  Subsystem2 : Subsystem
  Terminator{1..4,9} (5 alike) : Terminator
  Unary Minus : UnaryMinus
  Steering_Wheel_norm : Outport
  Acceleration_pedal : Outport  Port=2
  Brack_pedal : Outport  Port=3
  Button_1 : Outport  Port=4
  Button_2 : Outport  Port=5
  Button_3 : Outport  Port=6
  Button_4 : Outport  Port=7
  Right_Padel : Outport  Port=8
  Left_Padel : Outport  Port=9
  Button_5 : Outport  Port=10
  Button_6 : Outport  Port=11
  Button_7 : Outport  Port=12
  Button_8 : Outport  Port=13
  Button_9 : Outport  Port=14
  Button_10 : Outport  Port=15
  arrow_deg : Outport  Port=16
  DNR : Outport  Port=17
  wires:
  Demux2/15 -> Terminator9/1
  Data Type Conversion3/1 -> Gain1/1
  Data Type Conversion2/1 -> Gain/1
  Add/1 -> DNR/1
  Gain1/1 -> Add/2
  Gain/1 -> Add/1
  Unary Minus/1 -> Steering_Wheel_norm/1
  Other Input/1 -> arrow_deg/1
  Demux2/19 -> Button_10/1
  Demux2/18 -> Button_9/1
  Demux2/17 -> Button_8/1
  Demux2/16 -> Button_7/1
  Demux2/8 -> Button_5/1  "Shifter_Up"
  Demux2/7 -> Button_6/1  "Right_Button_3"
  Demux2/6 -> Left_Padel/1  "Right_Button_2"
  Demux2/5 -> Right_Padel/1  "Right_Button_1"
  Demux2/4 -> Button_4/1  "Left_Button_3"
  Demux2/3 -> Button_3/1  "Left_Button_2"
  Demux2/2 -> Button_2/1  "Left_Button_1"
  Demux2/1 -> MATLAB Function1/1(neutral), Button_1/1  "Left_Paddle"
  MATLAB Function/1(brake) -> Subsystem1/1(In1)
  Subsystem2/1(Out1) -> Acceleration_pedal/1
  MATLAB Function2/2(brake) -> ?  "Brake"
  Selector3/1 -> Gain4/1, MATLAB Function/1(accPedal)  "acc"
  Digital Input/1 -> Demux2/1
  Demux2/9 -> Terminator1/1  "Shifter_Down"
  Demux2/10 -> Terminator2/1
  Demux2/11 -> Terminator3/1
  Gain2/1 -> Unary Minus/1
  Demux2/12 -> Terminator4/1
  MATLAB Function1/2(backward_op) -> Data Type Conversion3/1, Memory/1
  MATLAB Function1/1(forward_op) -> Memory1/1, Data Type Conversion2/1
  Selector/1 -> MATLAB Function1/3(forward_ip)
  Selector1/1 -> MATLAB Function1/2(backward_ip)
  Memory/1 -> MATLAB Function1/5(backward_memo)
  Memory1/1 -> MATLAB Function1/4(forward_memo)
  Gain3/1 -> Brack_pedal/1
  Subsystem1/1(Out1) -> Gain3/1
  Gain4/1 -> Subsystem2/1(In1)
  Joystick Input1/2 -> Display1/1, Selector/1, Selector1/1
  Joystick Input1/1 -> Selector4/1, Selector3/1, Selector2/1
  Selector2/1 -> Gain2/1
  Selector4/1 -> MATLAB Function/2(brakePedal)

== system Model_Platform/Vehicle model/Vehicle dynamics/Forces_transformation ==
  note: this block is to produce the whole
      | forces and moments that is applied
      | on the car transformed to the vehicle
      | center of gravity CG
  velocity_of_car_absolute : Inport
  Slip_angle_of_velocity : Inport  Port=2
  Forces_on_x_from_wheel_mux(4) : Inport  Port=3
  Forces_on_y_from_wheel_mux(4) : Inport  Port=4
  Forces_on_z_from_wheel_mux(4) : Inport  Port=5
  Length_suspention(4) : Inport  Port=6
  Z0_mux(4) : Inport  Port=7
  Demux : Demux
  Force_of_Aerodynamics : Subsystem
  Moment _about _Z_axis_calculation : Subsystem
  Moment _about _x_axis_calculation : Subsystem
  Moment _about _y_axis_calculation : Subsystem
  Z1-->angles : Subsystem
  force acting in X direction : Subsystem
  force acting in Y direction : Subsystem
  force acting in Z direction : Subsystem
  inclination_effect_on_mass : Subsystem
  Force_acting_on_CG_in_x : Outport
  Force_acting_on_CG_in_Y : Outport  Port=2
  Moment _about _Z_axis : Outport  Port=3
  Force_acting_on_CG_in_z : Outport  Port=4
  Moment _about _X_axis : Outport  Port=5
  Moment _about _Y_axis : Outport  Port=6
  Mass*gravity_in_Z : Outport  Port=7
  wires:
  Z0_mux(4)/1 -> Z1-->angles/1(Z1(4))
  inclination_effect_on_mass/3(Fy_due_to_mass) -> force acting in Y direction/2(Force_From_Mass_Y)
  inclination_effect_on_mass/2(Fx_due_to_mass) -> force acting in X direction/2(Force_acting_in_x_from_mass)
  Z1-->angles/1(Roll_angel(z1)1) -> inclination_effect_on_mass/1(Roll_angle(z1))
  Z1-->angles/2(Pitch_angel(z1)) -> inclination_effect_on_mass/2(Pitch_angel(z1))
  Length_suspention(4)/1 -> Demux/1
  Force_of_Aerodynamics/1(Force_of_aerodynamics_in_X) -> force acting in X direction/3(Force_in_x_air)
  Demux/4 -> Moment _about _y_axis_calculation/6(Hight_Rear_Right), Moment _about _x_axis_calculation/6(Hight_Rear_Right)
  Demux/3 -> Moment _about _y_axis_calculation/5(Hight_Rear_Left), Moment _about _x_axis_calculation/5(Hight_Rear_Left)
  Demux/2 -> Moment _about _y_axis_calculation/4(Hight_Front_Right), Moment _about _x_axis_calculation/4(Hight_Front_Right)
  Demux/1 -> Moment _about _y_axis_calculation/3(Hight_Front_Left), Moment _about _x_axis_calculation/3(Hight_Front_Left)
  Moment _about _y_axis_calculation/1(Moment _about _Y_axis2) -> Moment _about _Y_axis/1
  inclination_effect_on_mass/1(FZ_due_to_mass) -> Mass*gravity_in_Z/1, force acting in Z direction/2(Force_Mass_Z)
  Moment _about _x_axis_calculation/1(Moment _about _X_axis1) -> Moment _about _X_axis/1
  force acting in Z direction/1(Force_acting_on_CG_in_z) -> Force_acting_on_CG_in_z/1
  Forces_on_z_from_wheel_mux(4)/1 -> Moment _about _y_axis_calculation/1(Forces_Z_Wheels), Moment _about _x_axis_calculation/1(Forces_Z_Wheels), force acting in Z direction/1(Forces_Z_Wheel)
  Forces_on_y_from_wheel_mux(4)/1 -> force acting in Y direction/1(Forces_Acting_In_Y_Wheels), Moment _about _Z_axis_calculation/2(Forces_Acting_in_Y_Wheels), Moment _about _x_axis_calculation/2(Forces_Y_Wheels)
  Forces_on_x_from_wheel_mux(4)/1 -> Moment _about _y_axis_calculation/2(Forces_X_Wheels), Moment _about _Z_axis_calculation/1(Forces_Acting_in_X_Wheels), force acting in X direction/1(Forces_Acting_In_X_Wheel)
  Slip_angle_of_velocity/1 -> Force_of_Aerodynamics/2(Slip_angle_of_velocity)
  velocity_of_car_absolute/1 -> Force_of_Aerodynamics/1(velocity_of_car_absolut)
  Moment _about _Z_axis_calculation/1(Moment _about _Z_axis) -> Moment _about _Z_axis/1
  force acting in Y direction/1(Force_acting_on_CG_in_Y) -> Force_acting_on_CG_in_Y/1
  force acting in X direction/1(Force_acting_on_CG_in_x) -> Force_acting_on_CG_in_x/1

== system Model_Platform/Vehicle model/Vehicle dynamics/Horizontal_Dyn ==
  note: in each one of these three blocks
      | only devision by mass or inertia
      | then integration is to be applied
      | as the force was derived and
      | transformed purely  to the CG
  note: through this block the displacement in
      | x and y and the yaw angle could be
      | developed to discribe the car movement
      | in the horizontal plan
  Force_acting_on_CG_in_x : Inport
  Force_acting_on_CG_in_y : Inport  Port=2
  Moment _about _Z_axis : Inport  Port=3
  vx[m|s] : Inport  Port=4
  Beta_Slip_Angle_calculation : Subsystem
  Terminator : Terminator
  about_z_axis : Subsystem
  in_x_direction : Subsystem
  in_y_direction : Subsystem
  reset : Subsystem
  reset1 : Subsystem
  Longitudinal_velocity_Vx : Outport
  Lateral_velocity_Vy_relative_to_car : Outport  Port=2
  "yaw " : Outport  Port=3
  Displacement_y_relative_to_car : Outport  Port=4
  Displacement_x_relative_to_car : Outport  Port=5
  Beta_Slip_Angle : Outport  Port=6
  ACC_x_relative_to_car : Outport  Port=7
  ACC_Y_relative_to_car : Outport  Port=8
  Yaw_rate_of_change : Outport  Port=9
  absolute_velocity_of_car : Outport  Port=10
  wires:
  reset1/1(Out1) -> in_y_direction/2(reset)
  reset/1(Out1) -> about_z_axis/2(reset)
  vx[m|s]/1 -> reset1/1(In1), reset/1(In1)
  in_y_direction/1(Lateral_Velocity_Vy) -> Beta_Slip_Angle_calculation/2(Longitudinal_Velocity_Vy), Lateral_velocity_Vy_relative_to_car/1
  about_z_axis/1(Yaw_Angular_ACC) -> Terminator/1
  about_z_axis/2(Yaw_angle_Velcity) -> Yaw_rate_of_change/1
  about_z_axis/3(Yaw_angle_(rad)) -> "yaw "/1
  Beta_Slip_Angle_calculation/2(absolute_velocity_of_car_with_direction) -> absolute_velocity_of_car/1
  Beta_Slip_Angle_calculation/1(Beta_Slip_Angle) -> Beta_Slip_Angle/1
  in_y_direction/2(Displacement_y) -> Displacement_y_relative_to_car/1
  in_y_direction/3(Acceleration_Ay) -> ACC_Y_relative_to_car/1
  in_x_direction/3(Acceleration_Ax) -> ACC_x_relative_to_car/1
  in_x_direction/2(Displacement_x) -> Displacement_x_relative_to_car/1
  in_x_direction/1(Longitudinal_Velocity_Vx) -> Beta_Slip_Angle_calculation/1(Longitudinal_Velocity_Vx), Longitudinal_velocity_Vx/1
  Moment _about _Z_axis/1 -> about_z_axis/1(Moment _about _Z_axis)
  Force_acting_on_CG_in_y/1 -> in_y_direction/1(Force_acting_on_CG_in_y)
  Force_acting_on_CG_in_x/1 -> in_x_direction/1(Force_acting_on_CG_in_x)

== system Model_Platform/Vehicle model/Vehicle dynamics/Output_Maping ==
  Velocity_Wheels_X[m|s] : Inport
  Velocity_Wheels_Y[m|s] : Inport  Port=2
  Force_Suspention : Inport  Port=3
  Vx_COG[m|s] : Inport  Port=4
  Vy_COG[m|s] : Inport  Port=5
  ax_COG[m|s2] : Inport  Port=6
  Wheel_FL_Steering_Angle[rad] : Inport  Port=7
  Wheel_FR_Steering_Angle[rad] : Inport  Port=8
  position_CoG_Global_Vector[m] : Inport  Port=9
  Oriantation_CoG_Vector[rad] : Inport  Port=10
  Yaw_Rate[rad|s] : Inport  Port=11
  Wheel_Steering_Angle_Left[rad] : Inport  Port=12
  Wheel_Steering_Angle_Right[rad] : Inport  Port=13
  Bus Creator : BusCreator  Inputs=2
  Bus Creator2 : BusCreator  Inputs=11
  Subsystem1 : Subsystem
  Velocity_Wheels_Maping_Block : Subsystem
  Vehicle_Dynamics : Outport
  wires:
  Wheel_Steering_Angle_Right[rad]/1 -> Bus Creator2/11  "Wheel_Steering_Angle_Right[rad]"
  Wheel_Steering_Angle_Left[rad]/1 -> Bus Creator2/10  "Wheel_Steering_Angle_Left[rad]"
  Yaw_Rate[rad|s]/1 -> Bus Creator2/9  "Yaw_Rate[rad|s]"
  Vy_COG[m|s]/1 -> Bus Creator2/4  "Vy_COG[m|s]"
  ax_COG[m|s2]/1 -> Bus Creator2/5  "ax_COG[m|s2]"
  Wheel_FR_Steering_Angle[rad]/1 -> Bus Creator/2
  Wheel_FL_Steering_Angle[rad]/1 -> Bus Creator/1
  Oriantation_CoG_Vector[rad]/1 -> Bus Creator2/8
  position_CoG_Global_Vector[m]/1 -> Bus Creator2/7
  Bus Creator2/1 -> Vehicle_Dynamics/1  "Vehicle_Dynamics"
  Velocity_Wheels_Y[m|s]/1 -> Velocity_Wheels_Maping_Block/2(Velocity_Wheels_Y[m|s])
  Velocity_Wheels_X[m|s]/1 -> Velocity_Wheels_Maping_Block/1(Velocity_Wheels_X[m|s])
  Vx_COG[m|s]/1 -> Bus Creator2/3
  Force_Suspention/1 -> Subsystem1/1(Force_Suspention)
  Bus Creator/1 -> Bus Creator2/6  "Wheel_angle[rad]"
  Subsystem1/1(Fz_Wheel[N]) -> Bus Creator2/2  "Fz_Wheel"
  Velocity_Wheels_Maping_Block/1(Velocity_Wheels[m|s]) -> Bus Creator2/1

== system Model_Platform/Vehicle model/Vehicle dynamics/Vertical_Dyn. ==
  Vertical_Force_CG : Inport
  Moment_X-axis_CG : Inport  Port=2
  Moment_Y-axis_CG : Inport  Port=3
  Mass*gravity_in_Z : Inport  Port=4
  Z0 : Inport  Port=5
  Invers_Trangnometric_conv : Subsystem
  Mass_Distribution : Subsystem
  Trangnometric_conv : Subsystem
  Vertical_movement : Subsystem
  suspention_System : Subsystem
  Vertical_Displacement_Z_CG : Outport
  Vertical_Displacement_Z_vehicle_corners(4) : Outport  Port=2
  pitch : Outport  Port=3
  Roll : Outport  Port=4
  Force_Suspention(4) : Outport  Port=5
  Length_Suspention(4) : Outport  Port=6
  Z1(4) : Outport  Port=7
  Vertical_Velocity_Z_CG[m|s] : Outport  Port=8
  wires:
  Vertical_movement/4(Vertical_Velocity_Z_CG[m|s]) -> Vertical_Velocity_Z_CG[m|s]/1
  Trangnometric_conv/1(Vertical_Displacement_Z_vehicle_corners(4)) -> suspention_System/1(Vertical_Displacement_Z2_vehicle_corners(4))
  Mass*gravity_in_Z/1 -> Mass_Distribution/1(Mass*gravity_in_Z)
  Invers_Trangnometric_conv/2(Roll_actual) -> Roll/1
  Invers_Trangnometric_conv/1(Vertical_Displacement_Z_CG_actual) -> Vertical_Displacement_Z_CG/1
  suspention_System/4(Vertical_Displacement_Z_vehicle_corners_actual(4)) -> Vertical_Displacement_Z_vehicle_corners(4)/1, Invers_Trangnometric_conv/1(Vertical_Displacement_Z_vehicle_corners_actual(4))
  suspention_System/3(Z1(4)) -> Z1(4)/1
  Z0/1 -> suspention_System/2(Vertical_Displacement_Z0(4))
  Mass_Distribution/1(Forces_Z_Mass) -> suspention_System/3(intial_force_from_mass_Wheels(4))
  suspention_System/2(Hight_Suspention(4)) -> Length_Suspention(4)/1
  suspention_System/1(Force_Suspention(4)) -> Force_Suspention(4)/1
  Vertical_movement/3(Roll) -> Trangnometric_conv/3(Roll)
  Vertical_movement/2(Pitch) -> Trangnometric_conv/2(Pitch)
  Vertical_movement/1(Vertical_Displacement_Z_CG) -> Trangnometric_conv/1(Vertical_Displacement_Z_CG)
  Moment_X-axis_CG/1 -> Vertical_movement/3(Moment_X-axis_CG)
  Moment_Y-axis_CG/1 -> Vertical_movement/2(Moment_Y-axis_CG)
  Vertical_Force_CG/1 -> Vertical_movement/1(Vertical_Force_CG)
  Invers_Trangnometric_conv/3(Pitch_actual) -> pitch/1

== system Model_Platform/Vehicle model/Vehicle dynamics/force_from_wheel_cordination_transformation ==
  note: this block is to analyze the
      | forces acting on the wheels
      |  coordination to find thier
      | components on the car coordination
      | -with respect to CAR XY-
      | and provides the angle of rotation
      | of each wheel due to ackermann
  steering_Angle_HMI_in_range[-1 1] : Inport
  force_from_wheel_fornt_left_in_x_relative_to_tire : Inport  Port=2
  force_from_wheel_fornt_right_in_x_relative_to_tire : Inport  Port=3
  force_from_wheel_rear_left_in_x_relative_to_tire : Inport  Port=4
  force_from_wheel_rear_right_in_x_relative_to_tire : Inport  Port=5
  force_from_wheel_fornt_left_in_y_relative_to_tire : Inport  Port=6
  force_from_wheel_fornt_right_in_y_relative_to_tire : Inport  Port=7
  force_from_wheel_rear_left_in_y_relative_to_tire : Inport  Port=8
  force_from_wheel_rear_right_in_y_relative_to_tire : Inport  Port=9
  Mux : Mux
  Mux1 : Mux
  Steer_model : Subsystem
  Forces_on_x_from_wheel_mux(4) : Outport
  Forces_on_y_from_wheel_mux(4) : Outport  Port=2
  angle_of_rotation_of_front_left_wheel : Outport  Port=3
  angle_of_rotation_of_front_right_wheel : Outport  Port=4
  wires:
  steering_Angle_HMI_in_range[-1 1]/1 -> Steer_model/1(Steering_Angle_HMI_[-1 1])
  Steer_model/6(FR_Angle) -> angle_of_rotation_of_front_right_wheel/1
  Steer_model/5(FL_Angle) -> angle_of_rotation_of_front_left_wheel/1
  Mux1/1 -> Forces_on_y_from_wheel_mux(4)/1
  Mux/1 -> Forces_on_x_from_wheel_mux(4)/1
  force_from_wheel_rear_right_in_y_relative_to_tire/1 -> Mux1/4
  force_from_wheel_rear_left_in_y_relative_to_tire/1 -> Mux1/3
  Steer_model/3(FLy) -> Mux1/1
  Steer_model/4(FRy) -> Mux1/2
  force_from_wheel_rear_right_in_x_relative_to_tire/1 -> Mux/4
  force_from_wheel_rear_left_in_x_relative_to_tire/1 -> Mux/3
  Steer_model/2(FRx) -> Mux/2
  Steer_model/1(FLx) -> Mux/1
  force_from_wheel_fornt_right_in_y_relative_to_tire/1 -> Steer_model/5(FRy_T)
  force_from_wheel_fornt_left_in_y_relative_to_tire/1 -> Steer_model/4(FLy_T)
  force_from_wheel_fornt_right_in_x_relative_to_tire/1 -> Steer_model/3(FRx_T)
  force_from_wheel_fornt_left_in_x_relative_to_tire/1 -> Steer_model/2(FLx_T)
